simulink model "Regulator_o_zmiennej_strukturze2"  (R2015a)
settings: Solver=ode45  StartTime=0.0  StopTime=100  FixedStep=0.01  RelTol=1e-3
libraries: simulink x3
settings Model: Creator=Student  LastModifiedBy=lenovo
settings DebuggingCC: UnderspecifiedInitializationDetection=Classic

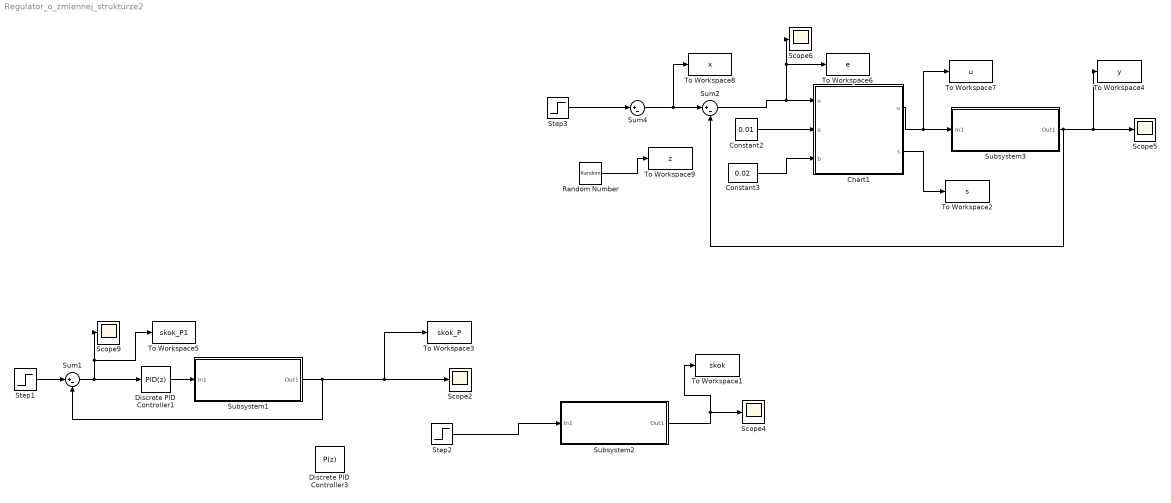
== system Regulator_o_zmiennej_strukturze2 ==
  Chart1 : Stateflow chart  TreatAsAtomicUnit=on
  Constant2 : Constant  Value=0.01
  Constant3 : Constant  Value=0.02
  Discrete PID Controller1 : simulink/Continuous/PID Controller  Controller=PID  TimeDomain=Discrete-time  SampleTime=1  IntegratorMethod=Forward Euler  FilterMethod=Forward Euler  Form=Parallel  UseFilter=on  ControllerParametersSource=internal  P=1.15918187545698  I=0.198333169990035  D=0.822383985307649  N=1.10226783906064  InitialConditionSource=internal  InitialConditionForIntegrator=0  InitialConditionForFilter=0  ExternalReset=none  LimitOutput=off  UpperSaturationLimit=inf  LowerSaturationLimit=-inf  LinearizeAsGain=off  AntiWindupMode=none  Kb=1  TrackingMode=off  Kt=1  PParamMin=[]  PParamMax=[]  IParamMin=[]  IParamMax=[]  DParamMin=[]  DParamMax=[]  NParamMin=[]  NParamMax=[]  KbParamMin=[]  KbParamMax=[]  KtParamMin=[]  KtParamMax=[]  POutMin=[]  POutMax=[]  IOutMin=[]  IOutMax=[]  DOutMin=[]  DOutMax=[]  NOutMin=[]  NOutMax=[]  KbOutMin=[]  KbOutMax=[]  KtOutMin=[]  KtOutMax=[]  IntegratorOutMin=[]  IntegratorOutMax=[]  FilterOutMin=[]  FilterOutMax=[]  SumOutMin=[]  SumOutMax=[]  SumI1OutMin=[]  SumI1OutMax=[]  SumI2OutMin=[]  SumI2OutMax=[]  SumI3OutMin=[]  SumI3OutMax=[]  SumDOutMin=[]  SumDOutMax=[]  SaturationOutMin=[]  SaturationOutMax=[]  IntegratorContinuousStateAttributes=''  IntegratorStateMustResolveToSignalObject=off  IntegratorRTWStateStorageClass=Auto  FilterContinuousStateAttributes=''  FilterStateMustResolveToSignalObject=off  FilterRTWStateStorageClass=Auto  DifferentiatorICPrevScaledInput=0  DifferentiatorOutMin=[]  DifferentiatorOutMax=[]
  Discrete PID Controller3 : simulink/Continuous/PID Controller  Controller=P  TimeDomain=Discrete-time  SampleTime=1  IntegratorMethod=Forward Euler  FilterMethod=Forward Euler  Form=Parallel  UseFilter=on  ControllerParametersSource=internal  P=1.49730031613405  I=0.178941537116669  D=2.4730817878  N=1.88002834107625  InitialConditionSource=internal  InitialConditionForIntegrator=0  InitialConditionForFilter=0  ExternalReset=none  LimitOutput=off  UpperSaturationLimit=inf  LowerSaturationLimit=-inf  LinearizeAsGain=off  AntiWindupMode=none  Kb=1  TrackingMode=off  Kt=1  PParamMin=[]  PParamMax=[]  IParamMin=[]  IParamMax=[]  DParamMin=[]  DParamMax=[]  NParamMin=[]  NParamMax=[]  KbParamMin=[]  KbParamMax=[]  KtParamMin=[]  KtParamMax=[]  POutMin=[]  POutMax=[]  IOutMin=[]  IOutMax=[]  DOutMin=[]  DOutMax=[]  NOutMin=[]  NOutMax=[]  KbOutMin=[]  KbOutMax=[]  KtOutMin=[]  KtOutMax=[]  IntegratorOutMin=[]  IntegratorOutMax=[]  FilterOutMin=[]  FilterOutMax=[]  SumOutMin=[]  SumOutMax=[]  SumI1OutMin=[]  SumI1OutMax=[]  SumI2OutMin=[]  SumI2OutMax=[]  SumI3OutMin=[]  SumI3OutMax=[]  SumDOutMin=[]  SumDOutMax=[]  SaturationOutMin=[]  SaturationOutMax=[]  IntegratorContinuousStateAttributes=''  IntegratorStateMustResolveToSignalObject=off  IntegratorRTWStateStorageClass=Auto  FilterContinuousStateAttributes=''  FilterStateMustResolveToSignalObject=off  FilterRTWStateStorageClass=Auto  DifferentiatorICPrevScaledInput=0  DifferentiatorOutMin=[]  DifferentiatorOutMax=[]
  Random Number : RandomNumber  Mean=0.05  Variance=0.01  SampleTime=1
  Scope{2,4..6,9} (5 alike) : Scope
      Scope2 settings: TimeRange=50  YMin=-0.2  YMax=1.6  SaveName=ScopeData2
      Scope4 settings: TimeRange=50  YMin=-0.2  YMax=1.6  SaveName=ScopeData2
      Scope5 settings: TimeRange=100  YMin=0.5811999999996471  YMax=0.581199999999775  SaveName=ScopeData4
      Scope6 settings: YMin=-1  YMax=2  SaveName=ScopeData5
      Scope9 settings: TimeRange=50  YMin=-0.2  YMax=1.6  SaveName=ScopeData8
  Step1 : Step  SampleTime=0
  Step2 : Step  SampleTime=0
  Step3 : Step  SampleTime=0
  Subsystem1 : Subsystem
  Subsystem2 : Subsystem
  Subsystem3 : Subsystem
  Sum1 : Sum  Inputs=|+-
  Sum2 : Sum  Inputs=|+-
  Sum4 : Sum  Inputs=|+-
  To Workspace1 : ToWorkspace  VariableName=skok  SaveFormat=Timeseries  SampleTime=-1
  To Workspace2 : ToWorkspace  VariableName=s  SaveFormat=Timeseries  SampleTime=-1
  To Workspace3 : ToWorkspace  VariableName=skok_P  SaveFormat=Timeseries  SampleTime=-1
  To Workspace4 : ToWorkspace  VariableName=y  SaveFormat=Timeseries  SampleTime=-1
  To Workspace5 : ToWorkspace  VariableName=skok_P1  SaveFormat=Timeseries  SampleTime=-1
  To Workspace6 : ToWorkspace  VariableName=e  SaveFormat=Timeseries  SampleTime=-1
  To Workspace7 : ToWorkspace  VariableName=u  SaveFormat=Timeseries  SampleTime=-1
  To Workspace8 : ToWorkspace  VariableName=x  SaveFormat=Timeseries  SampleTime=-1
  To Workspace9 : ToWorkspace  VariableName=z  SaveFormat=Timeseries  SampleTime=-1
  wires:
  Subsystem1/1(Out1) -> Sum1/2, To Workspace3/1, Scope2/1
  Step1/1 -> Sum1/1
  Sum1/1 -> Discrete PID Controller1/1, To Workspace5/1, Scope9/1
  Subsystem2/1(Out1) -> To Workspace1/1, Scope4/1
  Step2/1 -> Subsystem2/1(In1)
  Subsystem3/1(Out1) -> Sum2/2, To Workspace4/1, Scope5/1
  Chart1/1(u) -> To Workspace7/1, Subsystem3/1(In1)
  Sum2/1 -> To Workspace6/1, Scope6/1, Chart1/1(e)
  Constant3/1 -> Chart1/3(b)
  Constant2/1 -> Chart1/2(a)
  Discrete PID Controller1/1 -> Subsystem1/1(In1)
  Chart1/2(s) -> To Workspace2/1
  Step3/1 -> Sum4/1
  Sum4/1 -> To Workspace8/1, Sum2/1
  Random Number/1 -> To Workspace9/1

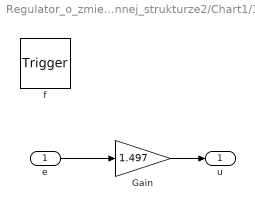
== system Regulator_o_zmiennej_strukturze2/Chart1/1.p ==
  e : Inport  OutDataTypeStr=double  PortDimensions=1
  f : TriggerPort  TriggerType=function-call
      settings: CopyFcn=Stateflow.SLINSF.SimulinkMan.removeBlockPreDeleteFcn  PreDeleteFcn=Stateflow.SLINSF.SimulinkMan.unsafePredeleteFcn
  Gain : Gain  Gain=1.497
  u : Outport
  wires:
  e/1 -> Gain/1
  Gain/1 -> u/1

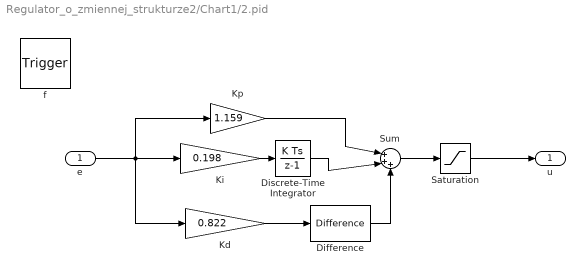
== system Regulator_o_zmiennej_strukturze2/Chart1/2.pid ==
  e : Inport  OutDataTypeStr=double  PortDimensions=1
  f : TriggerPort  TriggerType=function-call
      settings: CopyFcn=Stateflow.SLINSF.SimulinkMan.removeBlockPreDeleteFcn  PreDeleteFcn=Stateflow.SLINSF.SimulinkMan.unsafePredeleteFcn
  Difference : simulink/Discrete/Difference  ICPrevInput=0.0  InputProcessing=Inherited  OutMin=[]  OutMax=[]  OutDataType=fixdt(1, 16)  OutScaling=2^-10  DoSatur=off
  Discrete-Time Integrator : DiscreteIntegrator  InitialConditionSetting=State (most efficient)  SampleTime=-1
  Kd : Gain  Gain=0.822
  Ki : Gain  Gain=0.198
  Kp : Gain  Gain=1.159
  Saturation : Saturate  UpperLimit=1.1  LowerLimit=1
  Sum : Sum  Inputs=|+++
  u : Outport
  wires:
  Ki/1 -> Discrete-Time Integrator/1
  Kd/1 -> Difference/1
  Sum/1 -> Saturation/1
  Saturation/1 -> u/1
  Difference/1 -> Sum/3
  Discrete-Time Integrator/1 -> Sum/2
  Kp/1 -> Sum/1
  e/1 -> Kd/1, Kp/1, Ki/1

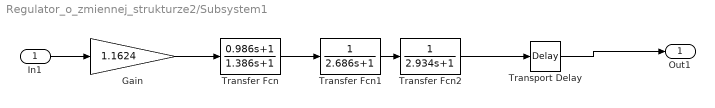
== system Regulator_o_zmiennej_strukturze2/Subsystem1 ==
  In1 : Inport
  Gain : Gain  Gain=1.1624
  Transfer Fcn : TransferFcn  Numerator=[0.986 1]  Denominator=[1.386 1]
  Transfer Fcn1 : TransferFcn  Denominator=[2.686 1]
  Transfer Fcn2 : TransferFcn  Denominator=[2.934 1]
  Transport Delay : TransportDelay  DelayTime=0.122  BufferSize=21504
  Out1 : Outport
  wires:
  Transfer Fcn1/1 -> Transfer Fcn2/1
  Transfer Fcn/1 -> Transfer Fcn1/1
  Transfer Fcn2/1 -> Transport Delay/1
  Transport Delay/1 -> Out1/1
  Gain/1 -> Transfer Fcn/1
  In1/1 -> Gain/1

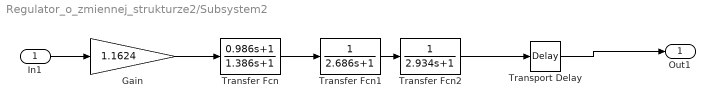
== system Regulator_o_zmiennej_strukturze2/Subsystem2 ==
  In1 : Inport
  Gain : Gain  Gain=1.1624
  Transfer Fcn : TransferFcn  Numerator=[0.986 1]  Denominator=[1.386 1]
  Transfer Fcn1 : TransferFcn  Denominator=[2.686 1]
  Transfer Fcn2 : TransferFcn  Denominator=[2.934 1]
  Transport Delay : TransportDelay  DelayTime=2.122  BufferSize=21504
  Out1 : Outport
  wires:
  Transfer Fcn1/1 -> Transfer Fcn2/1
  Transfer Fcn/1 -> Transfer Fcn1/1
  Transfer Fcn2/1 -> Transport Delay/1
  Transport Delay/1 -> Out1/1
  Gain/1 -> Transfer Fcn/1
  In1/1 -> Gain/1

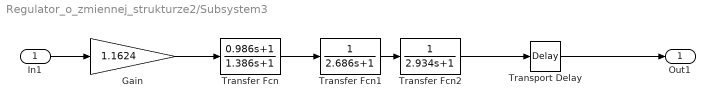
== system Regulator_o_zmiennej_strukturze2/Subsystem3 ==
  In1 : Inport
  Gain : Gain  Gain=1.1624
  Transfer Fcn : TransferFcn  Numerator=[0.986 1]  Denominator=[1.386 1]
  Transfer Fcn1 : TransferFcn  Denominator=[2.686 1]
  Transfer Fcn2 : TransferFcn  Denominator=[2.934 1]
  Transport Delay : TransportDelay  DelayTime=2.122  BufferSize=21504
  Out1 : Outport
  wires:
  Transfer Fcn1/1 -> Transfer Fcn2/1
  Transfer Fcn/1 -> Transfer Fcn1/1
  Transfer Fcn2/1 -> Transport Delay/1
  Transport Delay/1 -> Out1/1
  Gain/1 -> Transfer Fcn/1
  In1/1 -> Gain/1

== stateflow chart Regulator_o_zmiennej_strukturze2/Chart1 ==
  state 0
    entry: u=0;
    s=0;
  state 1
    entry: [u]=p(e)
    s=1;
    state u=p(e) [function]
  state 2
    entry: [u]=pid(e)
    s=2;
    state u=pid(e) [function]
  (default) -> 0
  2 -> 0 [order 1] : [e<a]
  0 -> 1 [order 1] : [e>a]
  0 -> 2 [order 2] : [e>b]
  1 -> 0 [order 2] : [e<a]
  2 -> 1 [order 2] : [e<b&&e>a ]
  1 -> 2 [order 1] : [e>b]
  data: u function_output; e function_input double size=1; e function_input double size=1; u function_output; e input; u output; a input; b input; s output
